simulink model "suspensionSimulink"  (R2015a)
settings: Solver=ode23t  StartTime=0.0  StopTime=10
PreLoadFcn:
  | load carParams
values from neighbouring files (symbols this model uses):
  b1 = 2500    [carParams.mat]
  b2 = 15000    [carParams.mat]
  k1 = 80000    [carParams.mat]
  k2 = 500000    [carParams.mat]
  mCar = 2500    [carParams.mat]
  mWheel = 200    [carParams.mat]
settings Model: Creator=scastro  LastModifiedBy=chahn
settings DataIOCC: LimitDataPoints=off  OutputTimes=0:0.001:60
settings SimscapeCC: SimscapeLogType=all  SimscapeLogDataHistory=10000

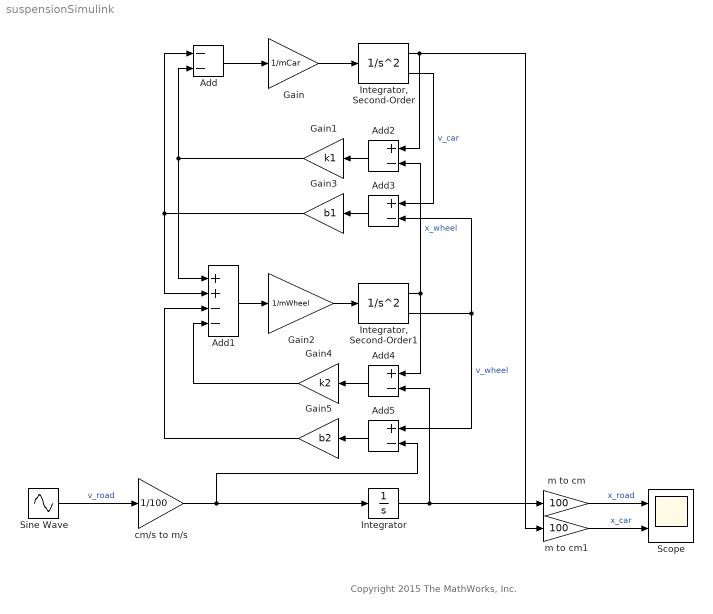
== system suspensionSimulink ==
  note: Copyright 2015 The MathWorks, Inc.
  Add : Sum  Inputs=--
  Add1 : Sum  Inputs=++--
  Add{2..5} (4 alike) : Sum  Inputs=+-
  Gain : Gain  Gain=1/mCar
  Gain1 : Gain  Gain=k1
  Gain2 : Gain  Gain=1/mWheel
  Gain3 : Gain  Gain=b1
  Gain4 : Gain  Gain=k2
  Gain5 : Gain  Gain=b2
  Integrator : Integrator
  "Integrator, Second-Order" : SecondOrderIntegrator
  "Integrator, Second-Order1" : SecondOrderIntegrator
  Scope : Scope  NumInputPorts=2
      settings: TimeRange=10  YMin=-4~-0.2  YMax=4~0.2
  Sine Wave : Sin  Amplitude=250  Frequency=100  Phase=pi/2  SampleTime=0
  cm/s to m/s : Gain  Gain=1/100
  m to cm : Gain  Gain=100
  m to cm1 : Gain  Gain=100
  wires:
  Integrator/1 -> Add4/2, m to cm/1
  cm/s to m/s/1 -> Add5/2, Integrator/1
  Gain/1 -> "Integrator, Second-Order"/1
  Add/1 -> Gain/1
  "Integrator, Second-Order"/1 -> m to cm1/1, Add2/1
  "Integrator, Second-Order"/2 -> Add3/1  "v_car"
  Gain2/1 -> "Integrator, Second-Order1"/1
  Add1/1 -> Gain2/1
  "Integrator, Second-Order1"/1 -> Add4/1, Add2/2  "x_wheel"
  "Integrator, Second-Order1"/2 -> Add3/2, Add5/1  "v_wheel"
  Add2/1 -> Gain1/1
  Add3/1 -> Gain3/1
  Gain1/1 -> Add1/1, Add/2
  Gain3/1 -> Add1/2, Add/1
  Add4/1 -> Gain4/1
  Gain4/1 -> Add1/4
  Add5/1 -> Gain5/1
  Gain5/1 -> Add1/3
  Sine Wave/1 -> cm/s to m/s/1  "v_road"
  m to cm/1 -> Scope/1  "x_road"
  m to cm1/1 -> Scope/2  "x_car"
